simulink model "BE6_7et8_auto"  (R2018b)
settings: Solver=VariableStepAuto  StartTime=0.0  StopTime=10  RelTol=1e-3
values from neighbouring files (symbols this model uses):
  A = [1  a1 a2]    [BE2_auto.m]    (also in BE6_7et8_auto.m = [l1 0 0; 0 0 1; l2 l3 0]; BE_synthese.m = [-alpha1 0; alpha1 -alpha2])
  B = [0 b1 b2]    [BE2_auto.m]    (also in BE6_7et8_auto.m = [l4; 0; 0]; BE_synthese.m = [sigma0; 0])
  C = [0 1 0]    [BE6_7et8_auto.m]    (also in BE_synthese.m = [0 1])
  F = place(A,B,roots)    [BE6_7et8_auto.m]    (also in BE_synthese.m = [Fe(1) Fe(2)])
  G = inv(-C*inv(A-B*F)*B)    [BE6_7et8_auto.m]    (also in BE_synthese.m = [Fe(3)])
settings Model: Creator=piffercg  LastModifiedBy=piffercg

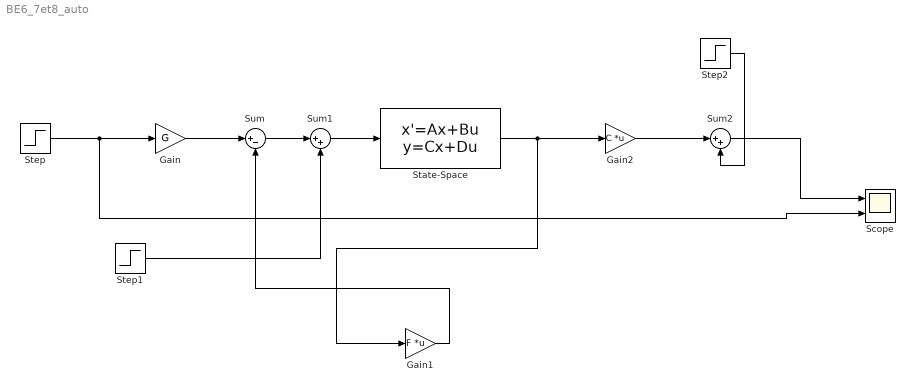
== system BE6_7et8_auto ==
  Gain : Gain  Gain=G
  Gain1 : Gain  Gain=F  Multiplication=Matrix(K*u)
  Gain2 : Gain  Gain=C  Multiplication=Matrix(K*u)
  Scope : Scope  NumInputPorts=2
  State-Space : StateSpace  A=A  B=B  C=eye(3)  D=zeros(3,1)  InitialCondition=0
  Step : Step  After=0.005  SampleTime=0
  Step1 : Step  Time=20  After=5  SampleTime=0
  Step2 : Step  Time=20  After=0.002  SampleTime=0
  Sum : Sum  Inputs=|+-
  Sum1 : Sum  Inputs=|++
  Sum2 : Sum  Inputs=|++
  wires:
  Step/1 -> Scope/2, Gain/1
  Gain/1 -> Sum/1
  State-Space/1 -> Gain1/1, Gain2/1
  Gain1/1 -> Sum/2
  Sum1/1 -> State-Space/1
  Sum/1 -> Sum1/1
  Step1/1 -> Sum1/2
  Gain2/1 -> Sum2/1
  Sum2/1 -> Scope/1
  Step2/1 -> Sum2/2
